simulink model "PressureControl_sim"  (R2021a)
settings: Solver=VariableStepAuto  StartTime=0.0  StopTime=3  RelTol=1e-3
undefined symbols (not defined in the file or in its folder): TF
settings Model: Creator=padlewsk  LastModifiedBy=padlewsk

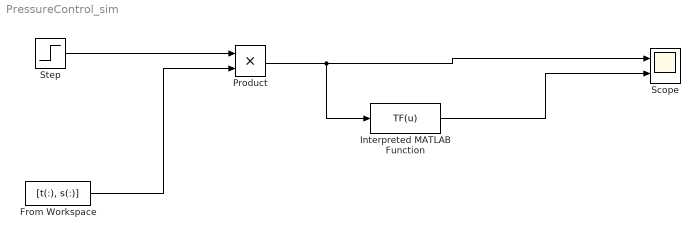
== system PressureControl_sim ==
  From Workspace : FromWorkspace  VariableName=[t(:), s(:)]  OutDataTypeStr=double  SampleTime=0.01  OutputAfterFinalValue=Holding final value
  Interpreted MATLAB Function : MATLABFcn  MATLABFcn=TF(u)
  Product : Product
  Scope : Scope  NumInputPorts=2
  Step : Step  Time=0.5  SampleTime=0
  wires:
  Step/1 -> Product/1
  From Workspace/1 -> Product/2
  Product/1 -> Interpreted MATLAB Function/1, Scope/1
  Interpreted MATLAB Function/1 -> Scope/2
